simulink model "Demo_Shore"  (R2014a)
settings: Solver=FixedStepDiscrete  SolverMode=SingleTasking  StartTime=0.0  StopTime=inf  FixedStep=0.01  RelTol=1e-3
PostLoadFcn:
  | h_RPStest = RPStest;
model workspace (MAT data in the model file):
  gtest = 0
undefined symbols (not defined in the file or in its folder): avert, avert_gaze_dirs_chance, avert_gaze_duration_factor, avert_head_frequency_factor, avert_head_speed, BML, BML1, BML2, bmlsL, bmlsM, bodyBusyFlag, clock, emotion_amount_factor, faceBusyFlag, fileID, GAZE_WIN, gazing, mutual_gaze_duration_factor, P, pose_chanc_factor, pose_chance_factor, pose_change_flag, pose_frequency_factor, pose_lean, pose_lean_flag, pose_selfAdaptor_chance_factor, pose_speed, pr, serial, STATE_BEFORE, STATE_GO, STATE_OVER, STATE_READY, Stateflow
libraries: simulink x23, instrumentlib x6, lib_affectiveChar_behavior x3, realtime_pacer_lib x2, lib_affectiveChar_input x1
(part 4 of 7)

== stateflow chart Demo_Shore/CharacterControl ==
  note: High Priority Tasks: Hand gesture for game
  state RPS_Scenario [parallel]
    settings: executionOrder=1
  note: Middle Priority Tasks: wave back at user and distance regulation
  state personalSpace_Controller [parallel]
    settings: executionOrder=5
  state wave_Controller [parallel]
    settings: executionOrder=7
  note: Low Priority Tasks: Idle gaze, pose and facial Expressions:
  state idlePose_Controller [parallel]
    settings: executionOrder=3
  state Gaze_Controller [parallel]
    settings: executionOrder=2
  state facialExpression_Controller [parallel]
    settings: executionOrder=4
  note: Parameters (can change
      | to seethe rangeof results)
      | -mutual_gaze_duration_factor
      | -avert_gaze_duration_factor
      | -avert_head_frequency_factor
      | -avert_head_speed(fast/slow/normal)
      | -avert_gaze_dirs_chance (down/up/normal)
      |
      | Inputs:(needed)
      | -faceAttendingFlag
      | -bodyAttendingFlag
  note: Parameters:
      | pose_selfAdaptor_chance_factor
      | pose_chance_factor
      | pose_frequency_factor
      | pose_speed(fast,slow,normal)
      | pose_lean(forward,backward,normal)
      |
      | Inputs:
      | -bodyAttendingFlag
  note: Parameters:
      |
      | Inputs:
      | -faceAttendingFlag
  note: Internal emotion/personality affects behavior modules (smile, gaze, pose)
  note: Instead of setting the factors directly in behavior or personality-emotion, added a module to centerlized and encapsulate all factors affecting behavior and their weights.
  state personality_Behavior_Factors [parallel]
    settings: executionOrder=9
  state emotion_Behavior_Factors [parallel]
    settings: executionOrder=10
  state custom_Behavior_Factors [parallel]
    settings: executionOrder=11
  note: Attention: if body or face is attending, no idle behavior are generated.
      | A queue is defined to priortize behaviors based on their importance.
  state attention_Controller [parallel]
    settings: executionOrder=8
  state sendBMLbyPriority [parallel]
    settings: executionOrder=6
    state sendH
      entry: BML=bmlsH(:,1);
      sendBML(BML);
      newBmlsH=removeQueue(bmlsH);
      bmlsH=newBmlsH;
    state init
      entry: n=encStr2Arr(' ');
      bmlsH=[n n n n n];
      bmlsM=[n n n n n];
      bmlsL=[n n n n n];
    state checkHighPriority
      entry:
      hEmpty=isEmptyQueue(bmlsH);
    state sendM
      entry: BML=bmlsM(:,1);
      sendBML(BML);
      newBmlsM= removeQueue(bmlsM);
      bmlsM=newBmlsM;
    state Mid
      entry:mEmpty=isEmptyQueue(bmlsM);
    state sendL
      entry: BML=bmlsL(:,1);
      sendBML(BML);
      newBmlsL= removeQueue(bmlsL);
      bmlsL=newBmlsL;
    state low
      entry:
      lEmpty=isEmptyQueue(bmlsL);
    note: Arrows' execution order is very importan here!
    state sendBML(In1) [function]
    sendH -> checkHighPriority
    checkHighPriority -> sendH [order 2] : [hEmpty~=1]
    (default) -> init
    init -> checkHighPriority
    checkHighPriority -> Mid [order 1] : [hEmpty==1]
    Mid -> checkHighPriority [order 4] : [mEmpty==1]
    sendM -> checkHighPriority [order 2]
    sendL -> checkHighPriority [order 3]
    low -> sendH [order 1] : [isEmptyQueue(bmlsH)~=1]
    Mid -> sendH [order 1] : [isEmptyQueue(bmlsH)~=1]
    sendM -> sendH [order 1] : [isEmptyQueue(bmlsH)~=1]
    sendL -> sendH [order 2] : [isEmptyQueue(bmlsH)~=1]
    Mid -> sendM [order 2] : [mEmpty~=1]
    Mid -> low [order 3] : [mEmpty==1]
    low -> Mid [order 4] : [lEmpty==1]
    low -> sendM [order 2] : [isEmptyQueue(bmlsM)~=1]
    sendL -> sendM [order 1] : [isEmptyQueue(bmlsM)~=1]
    low -> sendL [order 3] : [lEmpty~=1]
  data: In1 function_input double size=[1000 1]; bmls function_input; newBmls function_output; bmls function_input; empty function_output; emotion_amount_custom input double size=1; randArray input double size=[1,25]; poseArray input double size=[1,6]; gazeArray input double size=[1,6]; gameState output double size=1; inputUser input double size=1; bradHand output double size=1; userHand output double size=1; win output double size=1; temp local double size=1; diff local double size=1; uHand local double size=1; bHand local double size=1; bWinT output double size=1; uWinT output double size=1; randSmile local double size=1; boredom local double size=1; BOREDOM_THRESHOLD local double size=1; randAvertGazeChance local double size=1; randPoseChance local double size=1; interest local double size=1; r local double size=1; pa local double size=1; s local double size=1; randGazeDur local double size=1; P local double size=1 =0; smileN local double size=1; isSmiling input double size=1; body_isAttending input boolean size=1; face_isAttending input boolean size=1; avert local double size=1; GAZE_GUI local double size=1; GAZE_SOFTEYE local double size=1; GAZE_USER_HAND local double size=1; STATE_READY local double size=1 =0; STATE_GO local double size=1 =1; STATE_HAND local double size=1 =2; STATE_OVER local double size=1 =3; gazing local double size=1; GAZE_WIN local double size=1; randSlowPose local double size=1; STATE_BEFORE local double size=1 =4; STATE_RESULT local double size=1 =5; STATE_WAIT local double size=1 =6; HAPPY local double size=1 =4; SAD local double size=1 =4; CONTEMPT local double size=1 =4; BORED local double size=1 =4; FRUST local double size=1 =4; FEAR local double size=1 =4; IDLE local double size=1 =4; EXCITE local double size=1 =4; BML local double size=[1000,1]; pr local double size=1; t1 local; t2 local; round output double size=1; newBmlA local; fileID local double; xChangeFlag input boolean size=1; zChangeFlag input boolean size=1; isInvading input double size=1; inA input double size=1; handUp input double size=1; inV input double size=1; internalE input double size=1; personality input double size=1; BML2 local double size=[1000,1]; BML1 local double size=[1000,1]; t local double size=1; bodyBusyFlag local double size=1; n local double size=[1000,1]; bmlsL local double size=[1000,5]; hEmpty local double size=1; bmlsH local double size=[1000,5]; newBmlsH local double size=[1000,5]; newBmlsL local double size=[1000,5]; lEmpty local; newBmlsM local double size=[1000,5]; bmlsM local double size=[1000,5]; mEmpty local; avertH local double size=1; emoChange input boolean size=1; personalityChange input boolean size=1; faceBusyFlag local double size=1; personalityFlag input boolean size=1; vaFlag input boolean size=1; mutual_gaze_duration_factor local double size=1; avert_gaze_duration_factor local double size=1; avert_head_frequency_factor local double size=1; avert_gaze_dirs_chance local double size=1; avert_head_speed local double size=1; pose_chance_factor local double size=1; pose_selfAdaptor_chance_factor local double size=1; pose_frequency_factor local double size=1; pose_speed local double size=1; pose_lean local double size=1; pose_lean_flag local double size=1; pose_change_flag local double size=1; emotion_amount_factor local double size=[1,6]
  events: secs input RISING_EDGE_EVENT
  function newBmls=removeQueue(bmls):
    | function newBmls=removeQueue(bmls) 
    |     n=encStr2Arr(' ');
    |     newBmls=[n n n n n];
    |     newBmls(:,1)= bmls(:,2);
    |     newBmls(:,2)= bmls(:,3);
    |     newBmls(:,3)= bmls(:,4);
    |     newBmls(:,4)= bmls(:,5);
    |     newBmls(:,5)=encStr2Arr(' ');
  function empty=isEmptyQueue(bmls):
    | function empty=isEmptyQueue(bmls)
    | empty=1;
    | tempp=encStr2Arr(' ');
    | for i = 1:5
    |     if (isequal(bmls(:,i),tempp)==0)%there is a cell which is not equal to null
    |         empty=0;
    |         break
    |     end
    | end

== matlab function Demo_Shore/sendtoGUIFunction ==
  data: gameStatus input; bradHand input; userHand input; win input; bTotal input; uTotal input; gameNum input
function fcn(gameStatus, bradHand,userHand,win,bTotal,uTotal,gameNum)
%#codegen
setappdata(0,'gameStatus',gameStatus) 
setappdata(0,'bradHand',bradHand) 
setappdata(0,'userHand',userHand) 
setappdata(0,'win',win) 
setappdata(0,'uTotal',uTotal) 
setappdata(0,'bTotal',bTotal) 
setappdata(0,'gameNum',gameNum)

== matlab function Demo_Shore/readGlove/convertFunction ==
  data: u input; y output
function y = fcn(u)
%#codegen
%    paper=0; 'rock'=3;'scissors'=1;
%to 'paper'=1;'rock'=2;'scissors'=0;

if(u==0)
    u=1;
elseif(u==1)
    u=0;
elseif(u==3)
    u=2;
else 
    u=3;
end
y = u;

== stateflow chart Demo_Shore/CharacterControl/idlePose_Controller ==
  note: PERSONALITY:
      | -HN: self-touching and object manipulations, non-fluencies rigid posture and minimization of random movements, erect shoulder, cross legs Lean forward tenser
      | -LN:Lean backward reclining, head lean sideway or down
      | -High arousal: self and object adaptors, body tension and random trunk
      | For more info check Burgoon and Koper, 1984.
  note: -Ekman categorized hand poses to Emblems(e.g. hand shrug for helplessness or inability ; thumbs up), illustrators, Regulators, POINTS, Adaptors (self, alter-directed), spontaneousgests, attention-based gests
      | -Picking or squeezing part of the body is aggression against the self or aggression towards others temporarily displaced onto the self;
      | -covering the eye with a hand is relevant to preventing input, avoiding being seen, and shame
      | For more infor refer to Ekman (1972) Hand Movements.
  note: continously unpdate values based on change in valence-arousal
  note: The higher BOREDOMT (treshold), the lower chance of bored pose.
  note: Logically, personality parameters should only get calculated once. Since, here we change the personality dynamically during simulation,we calculate it in each loop.
  note: Problems with priortizing behaviors:
      |     1) When personality change, we want a few adjustments to happen e.g. agent's lean pose changes. The problem is system detects the change and set the flag to 1 and then again goes back to 0. If we dont check in stateflow exactly at that time we dont detect the change. that's why we need another flag that keeps the change till we do the personality based adjustment in behavior.After doing the adjustment we set that flag to zero.
      |     2) We can not use this for tracking if the body is busy at the time. When there is environmnet change agent reacts either by face or body (faceBusyFlag and bodyBusyFlag). We want to stop sending idle BML when they are busy. We need to check if flag is 1 excatly when we want to send the idle body or gaze BML.(if its a few milisec after or before it may not be busy. That's why we need attendChange module to set the flag to 1 for 10 sec after bodyBusy or faceBusy to avoid generating idle behavior in that period.
      |     3)problem also occures when the agent is at the middle of an idle pose/avert and needs to do interactive pose. It causes averted head+smile etc.
  state idlePoseGenerate [parallel]
    settings: executionOrder=1
    state stateInit
      entry:STATE_OVER=3;STATE_BEFORE=4;pose_lean_flag=0;
      STATE_READY=7;STATE_GO=1;gameState= 14;
      n=encStr2Arr(' ');bmlsL=[n n n n n];newBmlsL=[n n n n n];
    state leanChange
      entry:  pose_lean_flag=0;
      [P,BMLM]=weightshiftTable(pose_lean) ;
      newBmlsM=insertQueue(bmlsM,BMLM);
      bmlsM=newBmlsM;
    state stateRandomPose
      entry:
      randSlowPose=randArray(:,11);interest=BOREDOM_THRESHOLD-boredom;interest=1;
    state stateExtrovertPoseChance
      entry: randPoseChance=randi([0,round(interest*randSlowPose/pose_chance_factor)]);
    note: else
    note: else
    state poseCategoryChance1
      entry: randPR=randArray(:,20);
    state poseCategoryChance
      entry: randPR=randArray(:,20);
    note: else
    state selfAdaptorFast
      entry:
      [P,BMLl]=selfAdaptorTable(randArray(:,13)) ;
      newBmlsL=insertQueueLow(bmlsL,BMLl);
      bmlsL=newBmlsL;disp(decArr2Str(BMLl));
    state weightshiftFast
      entry:
      [P,BMLl]= weightshiftTable(randArray(:,21));
      newBmlsL=insertQueueLow(bmlsL,BMLl);
      bmlsL=newBmlsL;
    state weightshiftSlow
      entry:
      [P,BMLl]= weightshiftTable(randArray(:,22));
      newBmlsL=insertQueueLow(bmlsL,BMLl);
      bmlsL=newBmlsL;
    state selfAdaptorSlow
      entry:
      [P,BMLl]=selfAdaptorTable(randArray(:,14)) ;
      newBmlsL=insertQueueLow(bmlsL,BMLl);
      bmlsL=newBmlsL;disp(decArr2Str(BMLl));
    state weightshiftNormal
      entry:
      [P,BMLl]= weightshiftTable(randArray(:,22));
      newBmlsL=insertQueueLow(bmlsL,BMLl);
      bmlsL=newBmlsL;
    state selfAdaptorNormal
      entry:
      [P,BMLl]=selfAdaptorTable(randArray(:,14)) ;
      newBmlsL=insertQueueLow(bmlsL,BMLl);
      bmlsL=newBmlsL;disp(decArr2Str(BMLl));
    (default) -> stateInit
    stateInit -> stateRandomPose
    leanChange -> stateRandomPose : after(1,secs)
    stateRandomPose -> leanChange [order 1] : [pose_lean_flag==1]
    weightshiftFast -> stateRandomPose : after(pose_frequency_factor,secs)
    weightshiftSlow -> stateRandomPose : after(pose_frequency_factor,secs)
    weightshiftNormal -> stateRandomPose : after(pose_frequency_factor,secs)
    (junction 2) -> stateRandomPose [order 2]
    stateRandomPose -> stateExtrovertPoseChance [order 2]
    selfAdaptorNormal -> stateRandomPose : after(pose_frequency_factor,secs)
    selfAdaptorSlow -> stateRandomPose : after(pose_frequency_factor,secs)
    selfAdaptorFast -> stateRandomPose : after(pose_frequency_factor,secs)
    (junction 169) -> stateRandomPose [order 2]
    stateExtrovertPoseChance -> (junction 2) [order 2] : [pose_speed==2]
    stateExtrovertPoseChance -> (junction 169) [order 1] : [pose_speed==1]
    (junction 2) -> poseCategoryChance1 [order 1] : [[randPoseChance==1]&[ gameState~= STATE_GO]&[ gameState~= STATE_READY]]
    (junction 169) -> poseCategoryChance [order 1] : [[randPoseChance==1]&[ gameState~= STATE_GO]&[ gameState~= STATE_READY]]
    poseCategoryChance1 -> poseCategoryChance1 [order 2]
    poseCategoryChance -> poseCategoryChance [order 2]
    poseCategoryChance1 -> (junction 344) [order 1] : [bodyBusyFlag~=1]
    poseCategoryChance -> (junction 340) [order 1] : [bodyBusyFlag~=1]
    (junction 340) -> (junction 212) [order 1] : [randPR<=pose_selfAdaptor_chance_factor ]
    (junction 344) -> (junction 211) [order 1] : [randPR<=pose_selfAdaptor_chance_factor ]
    (junction 344) -> (junction 212) [order 2] : [randPR>pose_selfAdaptor_chance_factor ]
    (junction 340) -> (junction 211) [order 2] : [randPR>pose_selfAdaptor_chance_factor ]
    (junction 212) -> weightshiftNormal [order 3] : [pose_speed==0]
    (junction 212) -> weightshiftSlow [order 2] : [pose_speed==1]
    (junction 211) -> selfAdaptorNormal [order 3] : [pose_speed==0]
    (junction 211) -> selfAdaptorSlow [order 2] : [pose_speed==1]
    (junction 212) -> weightshiftFast [order 1] : [pose_speed==2]
    (junction 211) -> selfAdaptorFast [order 1] : [pose_speed==2]
  note: randSlowPose=randi(1,6)
  note: D10 for animation 8 which is hand on waist may not work with wave etc. Too long!
  note: else
  note: McNeill's gesture space sectors: the performance space in front of an actor is divided into three gesture space sections: Center-Center (CC), Center (C), and Periphery (P). CC is the central section directly in front of the chest, while subsequent sections (C and P) form spatial layers spreading outwards. low-warmth-low-competence performance consists of gestures mostly in the lower, center P region, while high-warmth-high-competence focuses mostly in the CC and C regions.
  data: pfreq function_output double size=1; v function_input double size=1; pChance function_output double size=1; ar function_input double size=1; p function_input double size=1; pCat function_output double size=1; pLean function_output double size=1; pfreq function_output double size=1; v function_input double size=1; pChance function_output double size=1; ar function_input double size=1; pfreqP function_input double size=1; pChanceP function_input double size=1; pCatP function_input double size=1; pCat function_output double size=1; pf function_output double size=1; p function_input double size=1; pL function_output double size=1; pC function_output double size=1; pCat function_output double size=1; bmlID function_input double; pr function_output double size=1; poseBML function_output double size=[1000,1]; pr function_output double size=1; bmlID function_input double; poseBML function_output double size=[1000,1]; pr function_output double size=1; bmlID function_input double; poseBML function_output double size=[1000,1]; p function_output double size=1; bmlID function_input double size=1; poseBML function_output double size=[1000,1]; bmls function_input double size=[1000,5]; myBML function_input double size=[1000,1]; newBmls function_output double size=[1000,5]; bmls function_input double size=[1000,5]; myBML function_input double size=[1000,1]; newBmls function_output double size=[1000,5]; boredom data_store_memory size=2; BOREDOM_THRESHOLD data_store_memory size=2; randSlowPose data_store_memory size=2; interest data_store_memory size=2; gameState output double size=1; randPoseChance data_store_memory size=1; STATE_OVER data_store_memory size=2; STATE_BEFORE data_store_memory size=2; STATE_READY data_store_memory size=2; inA input double size=1; inE input double size=1; HAPPY data_store_memory size=1 =4; SAD data_store_memory size=1 =4; CONTEMPT data_store_memory size=1 =4; BORED data_store_memory size=1 =4; FRUST data_store_memory size=1 =4; FEAR data_store_memory size=1 =4; IDLE data_store_memory size=1 =4; EXCITE data_store_memory size=1 =4; BML data_store_memory size=[256,1]; P data_store_memory; fileID data_store_memory; STATE_GO data_store_memory; bodyBusyFlag data_store_memory; BMLM local double size=[1000,1]; newBmlsL local double size=[1000,5]; bmlsL data_store_memory; n local; randArray input double size=[1,25]; personality input double size=1; randPR local; pPoseChance local; poseFreq local; leanPose local; inV input double size=1; pPoseChanceP local; poseFreqP local; pCatChance local; catChance local; personalityChange input boolean size=1; bmlsM data_store_memory; BMLl local double size=[1000,1]; newBmlsM local double size=[1000,5]; pChangeFlag local; faceBusyFlag data_store_memory; poseArray input double size=[1, 6]; pose_speed data_store_memory; pose_lean_flag data_store_memory; pose_lean data_store_memory; pose_frequency_factor data_store_memory; pose_chance_factor data_store_memory; pose_selfAdaptor_chance_factor data_store_memory; pose_change_flag data_store_memory
  events: secs input RISING_EDGE_EVENT
  function [pfreq,pChance,pCat,pLean]=setAffectParams(v,ar,p):
    | function [pfreq,pChance,pCat,pLean]=setAffectParams(v,ar,p)
    |      if(p==1) %HEHN
    |          pfreq=5;
    |          pLean=10;
    |          pChance=1;
    |          pCat=10;
    |      elseif(p==2)%LEHN
    |          pfreq=20;
    |          pLean=11;
    |          pChance=2;%to increase chance for HN
    |          pCat=10;
    |      elseif(p==3)%HELN
    |          pfreq=20;
    |          pLean=10;
    |          pChance=0.25;
    |          pCat=20;
    |      else%LELN
    |          pfreq=30;
    |          pLean=11;
    |          pChance=1;
    |          pCat=20;
    |      end
    |      
    |     if( ar>5)%A+
    |          pfreq=1.2*pfreq;
    |          pChance=1.1*pChance;
    |          pCat=pCat+2;
    |     end
    |     if(ar<-5)%A-
    |          pfreq=1.3*pfreq;
    |          pChance=1.1*pChance;
    |     end
    |     if(v>5)
    |         pCat=pCat-2;
    |     end
    |     if(v<-5)
    |         pCat=pCat+2;
    |     end
  function [pfreq,pChance,pCat]=setVAParams(v,ar,pfreqP,pChanceP,pCatP):
    | function [pfreq,pChance,pCat]=setVAParams(v,ar,pfreqP,pChanceP,pCatP)
    | if( ar>0)
    |      pfreq=1.2*pfreqP;
    |      pChance=1.1*pChanceP;
    |      pCat=pCatP+2;
    | else 
    |      pfreq=1.3*pfreqP;
    |      pChance=1.1*pChanceP;
    | end
    | if(v>0)
    |     pCat=pCatP-2;
    | else
    |     pCat=pCatP+2;
    | end
  function [pf,pL,pC,pCat]=setPersonalityParams(p):
    | function [pf,pL,pC,pCat]=setPersonalityParams(p)
    |  if(p==1) %HEHN
    |      pf=5;
    |      pL=10;
    |      pC=1;
    |      pCat=10;
    |  elseif(p==2)%LEHN
    |      pf=20;
    |      pL=11;
    |      pC=2;%to increase chance for HN
    |      pCat=10;
    |  elseif(p==3)%HELN
    |      pf=20;
    |      pL=10;
    |      pC=0.25;
    |      pCat=20;
    |  else%LELN
    |      pf=30;
    |      pL=11;
    |      pC=1;
    |      pCat=20;
    |  end
  function [pr,poseBML]=selfAdaptorTable(bmlID):
    | function [pr,poseBML]=selfAdaptorTable(bmlID)
    | 
    | aVarTruthTableCondition_1 = false;
    | aVarTruthTableCondition_2 = false;
    | aVarTruthTableCondition_3 = false;
    | aVarTruthTableCondition_4 = false;
    | aVarTruthTableCondition_5 = false;
    | aVarTruthTableCondition_6 = false;
    | aVarTruthTableCondition_7 = false;
    | aVarTruthTableCondition_8 = false;
    | aVarTruthTableCondition_9 = false;
    | aVarTruthTableCondition_10 = false;
    | aVarTruthTableCondition_11 = false;
    | aVarTruthTableCondition_12 = false;
    | aVarTruthTableCondition_13 = false;
    | aVarTruthTableCondition_14 = false;
    | aVarTruthTableCondition_15 = false;
    | aVarTruthTableCondition_16 = false;
    | aVarTruthTableCondition_17 = false;
    | aVarTruthTableCondition_18 = false;
    | aVarTruthTableCondition_19 = false;
    | aVarTruthTableCondition_20 = false;
    | 
    | 
    | 
    | aVarTruthTableCondition_1 = logical(bmlID==1);
    | 
    | 
    | aVarTruthTableCondition_2 = logical(bmlID==2);
    | 
    | 
    | aVarTruthTableCondition_3 = logical(bmlID==3);
    | 
    | 
    | aVarTruthTableCondition_4 = logical(bmlID==4);
    | 
    | 
    | aVarTruthTableCondition_5 = logical(bmlID==5);
    | 
    | 
    | aVarTruthTableCondition_6 = logical(bmlID==6);
    | 
    | 
    | aVarTruthTableCondition_7 = logical(bmlID==7);
    | 
    | 
    | aVarTruthTableCondition_8 = logical(bmlID==8);
    | 
    | 
    | aVarTruthTableCondition_9 = logical(bmlID==9);
    | 
    | 
    | aVarTruthTableCondition_10 = logical(bmlID==10);
    | 
    | 
    | aVarTruthTableCondition_11 = logical(bmlID==11);
    | 
    | 
    | aVarTruthTableCondition_12 = logical(bmlID==12);
    | 
    | 
    | aVarTruthTableCondition_13 = logical(bmlID==13);
    | 
    | 
    | aVarTruthTableCondition_14 = logical(bmlID==14);
    | 
    | 
    | aVarTruthTableCondition_15 = logical(bmlID==15);
    | 
    | 
    | aVarTruthTableCondition_16 = logical(bmlID==16);
    | 
    | 
    | aVarTruthTableCondition_17 = logical(bmlID==17);
    | 
    | 
    | aVarTruthTableCondition_18 = logical(bmlID==18);
    | 
    | 
    | aVarTruthTableCondition_19 = logical(bmlID==19);
    | 
    | 
    | aVarTruthTableCondition_20 = logical(bmlID==20);
    | 
    | if (aVarTruthTableCondition_1)
    |     aFcnTruthTableAction_1();
    | elseif (aVarTruthTableCondition_2)
    |     aFcnTruthTableAction_2();
    | elseif (aVarTruthTableCondition_3)
    |     aFcnTruthTableAction_3();
    | elseif (aVarTruthTableCondition_4)
    |     aFcnTruthTableAction_4();
    | elseif (aVarTruthTableCondition_5)
    |     aFcnTruthTableAction_5();
    | elseif (aVarTruthTableCondition_6)
    |     aFcnTruthTableAction_6();
    | elseif (aVarTruthTableCondition_7)
    |     aFcnTruthTableAction_7();
    | elseif (aVarTruthTableCondition_8)
    |     aFcnTruthTableAction_1();
    | elseif (aVarTruthTableCondition_9)
    |     aFcnTruthTableAction_2();
    | elseif (aVarTruthTableCondition_10)
    |     aFcnTruthTableAction_3();
    | elseif (aVarTruthTableCondition_11)
    |     aFcnTruthTableAction_11();
    | elseif (aVarTruthTableCondition_12)
    |     aFcnTruthTableAction_12();
    | elseif (aVarTruthTableCondition_13)
    |     aFcnTruthTableAction_13();
    | elseif (aVarTruthTableCondition_14)
    |     aFcnTruthTableAction_14();
    | elseif (aVarTruthTableCondition_15)
    |     aFcnTruthTableAction_15();
    | elseif (aVarTruthTableCondition_16)
    |     aFcnTruthTableAction_16();
    | elseif (aVarTruthTableCondition_17)
    |     aFcnTruthTableAction_17();
    | elseif (aVarTruthTableCondition_18)
    |     aFcnTruthTableAction_4();
    | elseif (aVarTruthTableCondition_19)
    |     aFcnTruthTableAction_5();
    | elseif (aVarTruthTableCondition_20)
    |     aFcnTruthTableAction_6();
    | else % Default
    |     aFcnTruthTableAction_1();
    | end
    | 
    | function aFcnTruthTableAction_1()
    | 
    | % WeightShiftFast
    | 
    | poseBML=encStr2Arr('<?xml version="1.0" ?><act><bml><animation name="ChrBrad@Idle01_WeightShift01" speed="2" /></bml></act>');pr=3;
    | 
    | function aFcnTruthTableAction_2()
    | 
    | % WeightShift2F
    | 
    | poseBML=encStr2Arr('<?xml version="1.0" ?><act><bml><animation name="ChrBrad@Idle01_WeightShift02" speed="2"/></bml></act>'); pr=3;
    | 
    | function aFcnTruthTableAction_3()
    | 
    | % ShoulderStretchUpDownF
    | 
    | poseBML=encStr2Arr('<?xml version="1.0" ?><act><bml><animation name="ChrBrad@Idle01_ShoulderStretch01" speed="2"/></bml></act>');pr=3;
    | 
    | function aFcnTruthTableAction_4()
    | 
    | % ScratchHeadF
    | 
    | poseBML=encStr2Arr('<?xml version="1.0" ?><act><bml><animation name="ChrBrad@Idle01_ScratchHeadLf01" speed="2"/></bml></act>'); pr=3;
    | 
    | function aFcnTruthTableAction_5()
    | 
    | % scratchtemple(head)F
    | 
    | poseBML=encStr2Arr('<?xml version="1.0" ?><act><bml><animation name="ChrBrad@Idle01_ScratchTempleLf01" speed="2"/></bml></act>'); pr=3;
    | 
    | function aFcnTruthTableAction_6()
    | 
    | % ScratchChestF
    | 
    | poseBML=encStr2Arr('<?xml version="1.0" ?><act><bml><animation name="ChrBrad@Idle01_ScratchChest01" speed="2"/></bml></act>');pr=3;
    | 
    | function aFcnTruthTableAction_7()
    | 
    | % SqueezeHand01F
    | 
    | poseBML=encStr2Arr('<?xml version="1.0" ?><act><bml><animation name="ChrBrad@Idle01_SqueezeHand01" speed="2" /></bml></act>');pr=3;
    | 
    | function aFcnTruthTableAction_8()
    | 
    | % brushCenterF
    | 
    | poseBML=encStr2Arr('<?xml version="1.0" ?><act><bml><gaze angle="10" direction="DOWNLEFT" sbm:joint-range="EYES NECK" sbm:time-hint="2" target="gazeTarget"/><gaze angle="20" direction="DOWNLEFT" sbm:joint-range="EYES" sbm:time-hint="2" target="gazeTarget"/><animation name="../data/ChrBrad/test_idle_brush_center.skm" speed="2"/></bml></act>'); pr=3;
    | 
    | function aFcnTruthTableAction_9()
    | 
    | % lookHandF
    | 
    | poseBML=encStr2Arr('<?xml version="1.0" ?><act><bml><gaze angle="10" direction="DOWNRIGHT" sbm:joint-range="EYES NECK" sbm:time-hint="2" target="gazeTarget"/><gaze angle="20" direction="DOWNRIGHT" sbm:joint-range="EYES" sbm:time-hint="2" target="gazeTarget"/><animation name="../data/ChrBrad/test_idle_hand_look.skm" speed="2"/></bml></act>'); pr=3;
    | 
    | function aFcnTruthTableAction_10()
    | 
    | % TouchHands01Slow-introvert
    | 
    | poseBML=encStr2Arr('<?xml version="1.0" ?><act><bml><animation name="ChrBrad@Idle01_TouchHands01" speed="0.8" /></bml></act>');pr=3;
    | 
    | function aFcnTruthTableAction_11()
    | 
    | % ScratchChestSlow
    | 
    | poseBML=encStr2Arr('<?xml version="1.0" ?><act><bml><animation name="ChrBrad@Idle01_ScratchChest01" speed="1"/></bml></act>');pr=3;
    | 
    | function aFcnTruthTableAction_12()
    | 
    | % WeightShiftSlow
    | 
    | poseBML=encStr2Arr('<?xml version="1.0" ?><act><bml><animation name="ChrBrad@Idle01_WeightShift01" speed="1" /></bml></act>');pr=3;
    | 
    | function aFcnTruthTableAction_13()
    | 
    | % scratchtempleSlow
    | 
    | poseBML=encStr2Arr('<?xml version="1.0" ?><act><bml><animation name="ChrBrad@Idle01_ScratchTempleLf01" speed="1" /></bml></act>');pr=3;
    | 
    | function aFcnTruthTableAction_14()
    | 
    | % SqueezeHandSlow
    | 
    | poseBML=encStr2Arr('<?xml version="1.0" ?><act><bml><animation name="ChrBrad@Idle01_SqueezeHand01" speed="1" /></bml></act>');pr=3;
    | 
    | function aFcnTruthTableAction_15()
    | 
    | % SqueezeHandSlowest
    | 
    | poseBML=encStr2Arr('<?xml version="1.0" ?><act><bml><animation name="ChrBrad@Idle01_SqueezeHand01" speed="0.7" /></bml></act>');pr=3;
    | 
    | function aFcnTruthTableAction_16()
    | 
    | % ShoulderStretchUpDownSlow
    | 
    | poseBML=encStr2Arr('<?xml version="1.0" ?><act><bml><animation name="ChrBrad@Idle01_ShoulderStretch01" speed="1"/></bml></act>');pr=3;
    | 
    | function aFcnTruthTableAction_17()
    | 
    | % WeightShift2Slow
    | 
    | poseBML=encStr2Arr('<?xml version="1.0" ?><act><bml><animation name="ChrBrad@Idle01_WeightShift02" speed="1"/></bml></act>'); pr=3;
    | 
    | function aFcnTruthTableAction_18()
    | 
    | % brushArmS
    | 
    | poseBML=encStr2Arr('<?xml version="1.0" ?><act><bml><gaze angle="20" direction="DOWNLEFT" sbm:joint-range="EYES NECK" sbm:time-hint="1" target="gazeTarget"/><gaze angle="30" direction="DOWNLEFT" sbm:joint-range="EYES" sbm:time-hint="1" target="gazeTarget"/><animation name="../data/ChrBrad/test_idle_brush.skm" speed="1"/></bml></act>'); pr=3;
    | 
    | function aFcnTruthTableAction_19()
    | 
    | % brushChestS
    | 
    | poseBML=encStr2Arr('<?xml version="1.0" ?><act><bml><gaze angle="10" direction="DOWNLEFT" sbm:joint-range="EYES NECK" sbm:time-hint="1" target="gazeTarget"/><gaze angle="20" direction="DOWNLEFT" sbm:joint-range="EYES" sbm:time-hint="1" target="gazeTarget"/><animation name="../data/ChrBrad/test_idle_brush_center.skm" speed="1"/></bml></act>'); pr=3;
    | 
    | function aFcnTruthTableAction_20()
    | 
    | % gazeAtHandS
    | 
    | poseBML=encStr2Arr('<?xml version="1.0" ?><act><bml><gaze angle="10" direction="DOWNRIGHT" sbm:joint-range="EYES NECK" sbm:time-hint="1" target="gazeTarget"/><gaze angle="20" direction="DOWNRIGHT" sbm:joint-range="EYES" sbm:time-hint="1" target="gazeTarget"/><animation name="../data/ChrBrad/test_idle_hand_look.skm" speed="1"/></bml></act>'); pr=3;
  function [pr,poseBML]=idlePoseBradOrigTable(bmlID):
    | function [pr,poseBML]=idlePoseBradOrigTable(bmlID)
    | 
    | aVarTruthTableCondition_1 = false;
    | aVarTruthTableCondition_2 = false;
    | aVarTruthTableCondition_3 = false;
    | aVarTruthTableCondition_4 = false;
    | aVarTruthTableCondition_5 = false;
    | aVarTruthTableCondition_6 = false;
    | aVarTruthTableCondition_7 = false;
    | aVarTruthTableCondition_8 = false;
    | aVarTruthTableCondition_9 = false;
    | aVarTruthTableCondition_10 = false;
    | aVarTruthTableCondition_11 = false;
    | aVarTruthTableCondition_12 = false;
    | aVarTruthTableCondition_13 = false;
    | aVarTruthTableCondition_14 = false;
    | aVarTruthTableCondition_15 = false;
    | aVarTruthTableCondition_16 = false;
    | aVarTruthTableCondition_17 = false;
    | aVarTruthTableCondition_18 = false;
    | aVarTruthTableCondition_19 = false;
    | aVarTruthTableCondition_20 = false;
    | aVarTruthTableCondition_21 = false;
    | aVarTruthTableCondition_22 = false;
    | 
    | 
    | 
    | aVarTruthTableCondition_1 = logical(bmlID==1);
    | 
    | 
    | aVarTruthTableCondition_2 = logical(bmlID==2);
    | 
    | 
    | aVarTruthTableCondition_3 = logical(bmlID==3);
    | 
    | 
    | aVarTruthTableCondition_4 = logical(bmlID==4);
    | 
    | 
    | aVarTruthTableCondition_5 = logical(bmlID==5);
    | 
    | 
    | aVarTruthTableCondition_6 = logical(bmlID==6);
    | 
    | 
    | aVarTruthTableCondition_7 = logical(bmlID==7);
    | 
    | 
    | aVarTruthTableCondition_8 = logical(bmlID==8);
    | 
    | 
    | aVarTruthTableCondition_9 = logical(bmlID==9);
    | 
    | 
    | aVarTruthTableCondition_10 = logical(bmlID==10);
    | 
    | 
    | aVarTruthTableCondition_11 = logical(bmlID==11);
    | 
    | 
    | aVarTruthTableCondition_12 = logical(bmlID==12);
    | 
    | 
    | aVarTruthTableCondition_13 = logical(bmlID==13);
    | 
    | 
    | aVarTruthTableCondition_14 = logical(bmlID==14);
    | 
    | 
    | aVarTruthTableCondition_15 = logical(bmlID==15);
    | 
    | 
    | aVarTruthTableCondition_16 = logical(bmlID==16);
    | 
    | 
    | aVarTruthTableCondition_17 = logical(bmlID==17);
    | 
    | 
    | aVarTruthTableCondition_18 = logical(bmlID==18);
    | 
    | 
    | aVarTruthTableCondition_19 = logical(bmlID==19);
    | 
    | 
    | aVarTruthTableCondition_20 = logical(bmlID==20);
    | 
    | 
    | aVarTruthTableCondition_21 = logical(bmlID==21);
    | 
    | 
    | aVarTruthTableCondition_22 = logical(bmlID==22);
    | 
    | if (aVarTruthTableCondition_1)
    |     aFcnTruthTableAction_1();
    | elseif (aVarTruthTableCondition_2)
    |     aFcnTruthTableAction_2();
    | elseif (aVarTruthTableCondition_3)
    |     aFcnTruthTableAction_3();
    | elseif (aVarTruthTableCondition_4)
    |     aFcnTruthTableAction_4();
    | elseif (aVarTruthTableCondition_5)
    |     aFcnTruthTableAction_4();
    | elseif (aVarTruthTableCondition_6)
    |     aFcnTruthTableAction_5();
    | elseif (aVarTruthTableCondition_7)
    |     aFcnTruthTableAction_6();
    | elseif (aVarTruthTableCondition_8)
    |     aFcnTruthTableAction_7();
    | elseif (aVarTruthTableCondition_9)
    |     aFcnTruthTableAction_3();
    | elseif (aVarTruthTableCondition_10)
    |     aFcnTruthTableAction_8();
    | elseif (aVarTruthTableCondition_11)
    |     aFcnTruthTableAction_9();
    | elseif (aVarTruthTableCondition_12)
    |     aFcnTruthTableAction_10();
    | elseif (aVarTruthTableCondition_13)
    |     aFcnTruthTableAction_11();
    | elseif (aVarTruthTableCondition_14)
    |     aFcnTruthTableAction_12();
    | elseif (aVarTruthTableCondition_15)
    |     aFcnTruthTableAction_13();
    | elseif (aVarTruthTableCondition_16)
    |     aFcnTruthTableAction_13();
    | elseif (aVarTruthTableCondition_17)
    |     aFcnTruthTableAction_14();
    | elseif (aVarTruthTableCondition_18)
    |     aFcnTruthTableAction_15();
    | elseif (aVarTruthTableCondition_19)
    |     aFcnTruthTableAction_16();
    | elseif (aVarTruthTableCondition_20)
    |     aFcnTruthTableAction_2();
    | elseif (aVarTruthTableCondition_21)
    |     aFcnTruthTableAction_17();
    | elseif (aVarTruthTableCondition_22)
    |     aFcnTruthTableAction_18();
    | else % Default
    |     aFcnTruthTableAction_9();
    | end
    | 
    | function aFcnTruthTableAction_1()
    | 
    | % ShoulderStretchUpDown
    | 
    | poseBML=encStr2Arr('<?xml version="1.0" ?><act><bml><animation name="ChrBrad@Idle01_ShoulderStretch01" speed="0.7"/></bml></act>');pr=3;
    | 
    | function aFcnTruthTableAction_2()
    | 
    | % scratchtemple(head)
    | 
    | poseBML=encStr2Arr('<?xml version="1.0" ?><act><bml><animation name="ChrBrad@Idle01_ScratchTempleLf01" speed="0.7"/></bml></act>'); pr=3;
    | 
    | function aFcnTruthTableAction_3()
    | 
    | % WeightShift2
    | 
    | poseBML=encStr2Arr('<?xml version="1.0" ?><act><bml><animation name="ChrBrad@Idle01_WeightShift02" speed="0.7"/></bml></act>'); pr=3;
    | 
    | function aFcnTruthTableAction_4()
    | 
    | % ScratchHead
    | 
    | poseBML=encStr2Arr('<?xml version="1.0" ?><act><bml><animation name="ChrBrad@Idle01_ScratchHeadLf01" speed="0.7"/></bml></act>'); pr=3;
    | 
    | function aFcnTruthTableAction_5()
    | 
    | % Idle01_ToIdle02
    | 
    | poseBML=encStr2Arr('<?xml version="1.0" ?><act><bml><animation name="ChrBrad@Idle01_ToIdle02" start="0"  ready="1" relax="4" stroke="3" end="6" speed="0.7"/></bml></act>');pr=3;
    | 
    | function aFcnTruthTableAction_6()
    | 
    | % ArmStretchHandsFW
    | 
    | poseBML=encStr2Arr('<?xml version="1.0" ?><act><bml><animation name="ChrBrad@Idle01_ArmStretch01"/></bml></act>');pr=3;
    | 
    | function aFcnTruthTableAction_7()
    | 
    | % ScratchChest
    | 
    | poseBML=encStr2Arr('<?xml version="1.0" ?><act><bml><animation name="ChrBrad@Idle01_ScratchChest01" speed="0.7"/></bml></act>');pr=3;
    | 
    | function aFcnTruthTableAction_8()
    | 
    | % HandsOnWaist
    | 
    | poseBML=encStr2Arr('<?xml version="1.0" ?><act><bml><animation name="ChrBrad@Idle01_ToIdle03" start="0" ready="2" stroke="3" stroke_end="5" relax="18" end="20" /></bml></act>');pr=3;
    | 
    | function aFcnTruthTableAction_9()
    | 
    | % SqueezeHand01
    | 
    | poseBML=encStr2Arr('<?xml version="1.0" ?><act><bml><animation name="ChrBrad@Idle01_SqueezeHand01" /></bml></act>');pr=3;
    | 
    | function aFcnTruthTableAction_10()
    | 
    | % TouchHands01
    | 
    | poseBML=encStr2Arr('<?xml version="1.0" ?><act><bml><animation name="ChrBrad@Idle01_TouchHands01" /></bml></act>');pr=3;
    | 
    | function aFcnTruthTableAction_11()
    | 
    | % WeightShift
    | 
    | poseBML=encStr2Arr('<?xml version="1.0" ?><act><bml><animation name="ChrBrad@Idle01_WeightShift01" /></bml></act>');pr=3;;
    | 
    | function aFcnTruthTableAction_12()
    | 
    | % ScratchChestSlow
    | 
    | poseBML=encStr2Arr('<?xml version="1.0" ?><act><bml><animation name="ChrBrad@Idle01_ScratchChest01" speed="0.5"/></bml></act>');pr=3;
    | 
    | function aFcnTruthTableAction_13()
    | 
    | % WeightShiftSlow
    | 
    | poseBML=encStr2Arr('<?xml version="1.0" ?><act><bml><animation name="ChrBrad@Idle01_WeightShift01" speed="0.5" /></bml></act>');pr=3;
    | 
    | function aFcnTruthTableAction_14()
    | 
    | % scratchtempleSlow
    | 
    | poseBML=encStr2Arr('<?xml version="1.0" ?><act><bml><animation name="ChrBrad@Idle01_ScratchTempleLf01" speed="0.5" /></bml></act>');pr=3;
    | 
    | function aFcnTruthTableAction_15()
    | 
    | % SqueezeHandSlow
    | 
    | poseBML=encStr2Arr('<?xml version="1.0" ?><act><bml><animation name="ChrBrad@Idle01_SqueezeHand01" speed="0.5" /></bml></act>');pr=3;
    | 
    | function aFcnTruthTableAction_16()
    | 
    | % SqueezeHandSlowest
    | 
    | poseBML=encStr2Arr('<?xml version="1.0" ?><act><bml><animation name="ChrBrad@Idle01_SqueezeHand01" speed="0.2" /></bml></act>');pr=3;
    | 
    | function aFcnTruthTableAction_17()
    | 
    | % ShoulderStretchUpDownSlow
    | 
    | poseBML=encStr2Arr('<?xml version="1.0" ?><act><bml><animation name="ChrBrad@Idle01_ShoulderStretch01" speed="0.5"/></bml></act>');pr=3;
    | 
    | function aFcnTruthTableAction_18()
    | 
    | % ScratchHeadSlow
    | 
    | poseBML=encStr2Arr('<?xml version="1.0" ?><act><bml><animation name="ChrBrad@Idle01_ScratchHeadLf01" speed="0.5" /></bml></act>');pr=3;
  function [pr,poseBML]=weightshiftTable(bmlID):
    | function [pr,poseBML]=weightshiftTable(bmlID)
    | 
    | aVarTruthTableCondition_1 = false;
    | aVarTruthTableCondition_2 = false;
    | aVarTruthTableCondition_3 = false;
    | aVarTruthTableCondition_4 = false;
    | aVarTruthTableCondition_5 = false;
    | aVarTruthTableCondition_6 = false;
    | aVarTruthTableCondition_7 = false;
    | aVarTruthTableCondition_8 = false;
    | aVarTruthTableCondition_9 = false;
    | aVarTruthTableCondition_10 = false;
    | aVarTruthTableCondition_11 = false;
    | 
    | 
    | 
    | aVarTruthTableCondition_1 = logical(bmlID==1);
    | 
    | 
    | aVarTruthTableCondition_2 = logical(bmlID==2);
    | 
    | 
    | aVarTruthTableCondition_3 = logical(bmlID==3);
    | 
    | % looks bad
    | 
    | aVarTruthTableCondition_4 = logical(bmlID==4);
    | 
    | 
    | aVarTruthTableCondition_5 = logical(bmlID==5);
    | 
    | 
    | aVarTruthTableCondition_6 = logical(bmlID==6);
    | 
    | 
    | aVarTruthTableCondition_7 = logical(bmlID==7);
    | 
    | 
    | aVarTruthTableCondition_8 = logical(bmlID==8);
    | 
    | 
    | aVarTruthTableCondition_9 = logical(bmlID==9);
    | 
    | 
    | aVarTruthTableCondition_10 = logical(bmlID==10);
    | 
    | 
    | aVarTruthTableCondition_11 = logical(bmlID==11);
    | 
    | if (aVarTruthTableCondition_1)
    |     aFcnTruthTableAction_1();
    | elseif (aVarTruthTableCondition_2)
    |     aFcnTruthTableAction_2();
    | elseif (aVarTruthTableCondition_3)
    |     aFcnTruthTableAction_3();
    | elseif (aVarTruthTableCondition_4)
    |     aFcnTruthTableAction_1();
    | elseif (aVarTruthTableCondition_5)
    |     aFcnTruthTableAction_5();
    | elseif (aVarTruthTableCondition_6)
    |     aFcnTruthTableAction_6();
    | elseif (aVarTruthTableCondition_7)
    |     aFcnTruthTableAction_7();
    | elseif (aVarTruthTableCondition_8)
    |     aFcnTruthTableAction_8();
    | elseif (aVarTruthTableCondition_9)
    |     aFcnTruthTableAction_9();
    | elseif (aVarTruthTableCondition_10)
    |     aFcnTruthTableAction_10();
    | elseif (aVarTruthTableCondition_11)
    |     aFcnTruthTableAction_11();
    | else % Default
    |     aFcnTruthTableAction_2();
    | end
    | 
    | function aFcnTruthTableAction_1()
    | 
    | % ShoulderStretchUpDownFast-Extrovert
    | 
    | poseBML=encStr2Arr('<?xml version="1.0" ?><act><bml><animation name="ChrBrad@Idle01_ShoulderStretch01" speed="2"/></bml></act>');pr=3;
    | 
    | function aFcnTruthTableAction_2()
    | 
    | % WeightShiftFast-HELN
    | 
    | poseBML=encStr2Arr('<?xml version="1.0" ?><act><bml><animation name="ChrBrad@Idle01_WeightShift01" speed="2"/></bml></act>');pr=3;;
    | 
    | function aFcnTruthTableAction_3()
    | 
    | % Idle01_ToIdle02Fast-HELN
    | 
    | poseBML=encStr2Arr('<?xml version="1.0" ?><act><bml><animation name="ChrBrad@Idle01_ToIdle02" speed="2"/></bml></act>');pr=4;
    | 
    | function aFcnTruthTableAction_4()
    | 
    | % HandsOnWaistFast-HELN-look bad
    | 
    | poseBML=encStr2Arr('<?xml version="1.0" ?><act><bml><animation name="ChrBrad@Idle01_ToIdle03" start="0" ready="1" stroke="2" stroke_end="3" relax="18" end="20" /></bml></act>');pr=4;
    | 
    | function aFcnTruthTableAction_5()
    | 
    | % ArmStretchHandsFWFast-HELN
    | 
    | poseBML=encStr2Arr('<?xml version="1.0" ?><act><bml><animation name="ChrBrad@Idle01_ArmStretch01" speed="2"/></bml></act>');pr=3;
    | 
    | function aFcnTruthTableAction_6()
    | 
    | % WeightShift2Fast-HELN
    | 
    | poseBML=encStr2Arr('<?xml version="1.0" ?><act><bml><animation name="ChrBrad@Idle01_WeightShift02" speed="2"/></bml></act>'); pr=3;
    | 
    | function aFcnTruthTableAction_7()
    | 
    | % WeightShift2Slow-LELN
    | 
    | poseBML=encStr2Arr('<?xml version="1.0" ?><act><bml><animation name="ChrBrad@Idle01_WeightShift02" speed="0.5"/></bml></act>'); pr=3;
    | 
    | function aFcnTruthTableAction_8()
    | 
    | % WeightShiftSlow-LELN
    | 
    | poseBML=encStr2Arr('<?xml version="1.0" ?><act><bml><animation name="ChrBrad@Idle01_WeightShift01" speed="0.5" /></bml></act>');pr=3;
    | 
    | function aFcnTruthTableAction_9()
    | 
    | % ShoulderStretchUpDownSlow-LELN
    | 
    | poseBML=encStr2Arr('<?xml version="1.0" ?><act><bml><animation name="ChrBrad@Idle01_ShoulderStretch01" speed="0.5"/></bml></act>');pr=3;
    | 
    | function aFcnTruthTableAction_10()
    | 
    | % extrovertLeanBack
    | 
    | poseBML=encStr2Arr('<?xml version="1.0" ?><act><bml><gaze angle="5" direction="UP" sbm:joint-range="HEAD CHEST" sbm:time-hint="2" target="gazeTarget"/></bml></act>'); pr=3;
    | 
    | function aFcnTruthTableAction_11()
    | 
    | % introvertLeanFW
    | 
    | poseBML=encStr2Arr('<?xml version="1.0" ?><act><bml><gaze angle="5" direction="DOWN" sbm:joint-range="HEAD CHEST" sbm:time-hint="2" target="gazeTarget"/></bml></act>'); pr=3;
  function [p,poseBML]=walkInvadingTable(bmlID):
    | function [p,poseBML]=walkInvadingTable(bmlID)
    | 
    | aVarTruthTableCondition_1 = false;
    | aVarTruthTableCondition_2 = false;
    | aVarTruthTableCondition_3 = false;
    | aVarTruthTableCondition_4 = false;
    | 
    | 
    | % n
    | 
    | aVarTruthTableCondition_1 = logical(bmlID==1);
    | 
    | % b
    | 
    | aVarTruthTableCondition_2 = logical(bmlID==2);
    | 
    | % f
    | 
    | aVarTruthTableCondition_3 = logical(bmlID==3);
    | 
    | % HN
    | 
    | aVarTruthTableCondition_4 = logical(bmlID==4);
    | 
    | if (aVarTruthTableCondition_1)
    |     aFcnTruthTableAction_1();
    | elseif (aVarTruthTableCondition_2)
    |     aFcnTruthTableAction_2();
    | elseif (aVarTruthTableCondition_3)
    |     aFcnTruthTableAction_3();
    | elseif (aVarTruthTableCondition_4)
    |     aFcnTruthTableAction_4();
    | else % Default
    |     aFcnTruthTableAction_1();
    | end
    | 
    | function aFcnTruthTableAction_1()
    | 
    | % Neutral
    | 
    | poseBML=encStr2Arr( '<?xml version="1.0" ?><act><bml><locomotion manner="walk" facing="camera"  sbm:accel="0.5" sbm:scootaccel="50" target="0 0"/></bml></act>');p=1;
    | 
    | function aFcnTruthTableAction_2()
    | 
    | % Back
    | 
    | poseBML=encStr2Arr( '<?xml version="1.0" ?><act><bml><locomotion manner="walk"  sbm:accel="0.5" sbm:scootaccel="50" facing="camera" target="0 -0.6"/></bml></act>');p=1;
    | 
    | function aFcnTruthTableAction_3()
    | 
    | % Forward
    | 
    | poseBML=encStr2Arr( '<?xml version="1.0" ?><act><bml><locomotion manner="walk" facing="camera"  sbm:accel="0.5" sbm:scootaccel="50" target="0 0.6"/></bml></act>');p=1;
    | 
    | function aFcnTruthTableAction_4()
    | 
    | % NeutralHead
    | 
    | poseBML=encStr2Arr('<?xml version="1.0" ?><act><bml><gaze target="camera" sbm:joint-range="EYES NECK" sbm:time-hint="1.5"/></bml></act>');p=1;
  function newBmls =insertQueueLow(bmls,myBML):
    | function newBmls =insertQueueLow(bmls,myBML)
    |     full=1;
    |     t=encStr2Arr(' ');
    |     newBmls=[t t t t t];
    |     for i = 1:5
    |         if (isequal(bmls(:,i),t))
    |             %add to end of the queue where its empty
    |             bmls(:,i)=myBML;
    |             full=0;
    |             break
    |         end
    |     end
    |     if(full~=0)
    |             %if queue full, shift all elements to left which removes the first one, then add to end
    |             bmls(:,1)= bmls(:,2);
    |             bmls(:,2)= bmls(:,3);
    |             bmls(:,3)= bmls(:,4);
    |             bmls(:,5)=myBML;
    |     end
    |     newBmls=bmls;
  function newBmls =insertQueue(bmls,myBML):
    | function newBmls =insertQueue(bmls,myBML)
    |     full=1;
    |     t=encStr2Arr(' ');
    |     newBmls=[t t t t t];
    |     for i = 1:5
    |         if (isequal(bmls(:,i),t))
    |             %add to end of the queue where its empty
    |             bmls(:,i)=myBML;
    |             full=0;
    |             break
    |         end
    |     end
    |     if(full~=0)
    |             %if queue full, shift all elements to left which removes the first one, then add to end
    |             bmls(:,1)= bmls(:,2);
    |             bmls(:,2)= bmls(:,3);
    |             bmls(:,3)= bmls(:,4);
    |             bmls(:,5)=myBML;
    |     end
    |     newBmls=bmls;

== matlab function Demo_Shore/moveFWTable ==
  data: z input; y output
function y = fcn(z)

aVarTruthTableCondition_1 = false;
aVarTruthTableCondition_2 = false;
aVarTruthTableCondition_3 = false;
aVarTruthTableCondition_4 = false;


% too far

aVarTruthTableCondition_1 = logical(z >= 220);

% too close

aVarTruthTableCondition_2 = logical(z < 150 && z~=0);

% properSpace

aVarTruthTableCondition_3 = logical(z>=150 && z<220);

% no value

aVarTruthTableCondition_4 = logical(z==0);

if (aVarTruthTableCondition_1)
    aFcnTruthTableAction_1();
elseif (aVarTruthTableCondition_2)
    aFcnTruthTableAction_2();
elseif (aVarTruthTableCondition_3)
    aFcnTruthTableAction_3();
elseif (aVarTruthTableCondition_4)
    aFcnTruthTableAction_4();
else % Default
    aFcnTruthTableAction_4();
end

function aFcnTruthTableAction_1()

% too far

y = 2;

function aFcnTruthTableAction_2()

% too close

y = 1;

function aFcnTruthTableAction_3()

% properSpace

y = 0;

function aFcnTruthTableAction_4()

% no value

y = 3;

== matlab function Demo_Shore/gazeTable ==
  data: x input; y output
function y = fcn(x)

aVarTruthTableCondition_1 = false;
aVarTruthTableCondition_2 = false;


% moved left

aVarTruthTableCondition_1 = logical(x > 50);

% moved right

aVarTruthTableCondition_2 = logical(x < -50);

if (aVarTruthTableCondition_1)
    aFcnTruthTableAction_1();
elseif (aVarTruthTableCondition_2)
    aFcnTruthTableAction_2();
else % Default
    aFcnTruthTableAction_3();
end

function aFcnTruthTableAction_1()

% moved left

y = 1;

function aFcnTruthTableAction_2()

% moved right

y = 2;

function aFcnTruthTableAction_3()

% proper place

y = 0;
